simulink model "SIRAu_PI_vit"  (Simulink 8.7)
settings: Solver=ode5  StartTime=0.0  StopTime=Temps_manip  FixedStep=TE  RelTol=1e-3
values from neighbouring files (symbols this model uses):
  Kmes = 10.7e-3    (= 0.0107)    [Param_PI_Vit.m]
  Kp = Tn/Ti    (= 2.64498624343)    [Param_PI_Vit.m]    (also in labo4.m = wc * sqrt(1+(wc*tau_ele)^2) * Ti / K_total)
  Td = 0    [Param_PI_Vit.m]
  TE = 1e-3    (= 0.001)    [Param_PI_Vit.m]
  Ti = 2 * Ks * T2    (= 0.0030245904)    [Param_PI_Vit.m]    (also in labo4.m = 0.008)
libraries: xpcnilib x2, simulink x1, simulink_extras x1
settings Model: Creator=allenbach  LastModifiedBy=jeremy.olivier
settings SolverCC: EnableConcurrentExecution=on  PositivePriorityOrder=on  AutoInsertRateTranBlk=on
settings DataIOCC: LimitDataPoints=off  SignalLoggingSaveFormat=ModelDataLogs
settings OptimizationCC: BlockReduction=off  OptimizeBlockIOStorage=off  BufferReuse=off  GlobalBufferReuse=off  ExpressionFolding=off  ExpressionDepthLimit=2147483647  LocalBlockOutputs=off
settings DebuggingCC: SolverPrmCheckMsg=warning  FcnCallInpInsideContextMsg=UseLocalSettings  StateNameClashWarn=warning
settings HardwareCC: ProdIntDivRoundTo=Zero  ProdEndianess=LittleEndian  ProdLongLongMode=on  ProdHWDeviceType=Generic->32-bit x86 compatible
settings RTWCC: SystemTargetFile=slrt.tlc  TemplateMakefile=slrt_default_tmf  Description=Simulink Real-Time  RTWCompilerOptimization=on
settings SimulinkRealTimeCC: GeneratePreprocessorConditionals=Disable all  RL32LogBufSizeModifier=300000

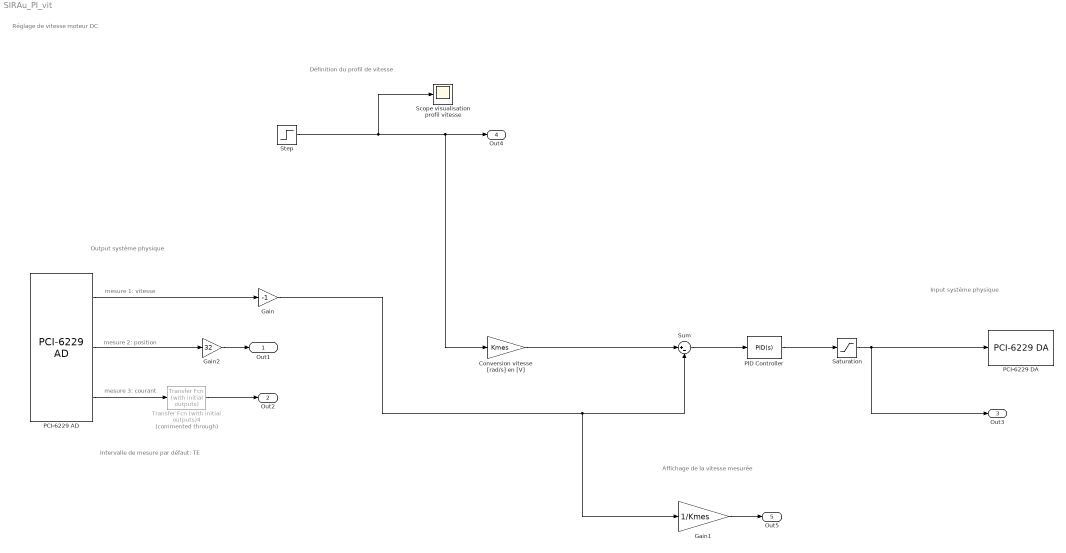
== system SIRAu_PI_vit ==
  note: Affichage de la vitesse mesurée
  note: Output système physique
  note: Input système physique
  note: Définition du profil de vitesse
  note: mesure 1: vitesse
  note: Réglage de vitesse moteur DC
  note: mesure 3: courant
  note: mesure 2: position
  note: Intervalle de mesure par défaut: TE
  Conversion vitesse [rad/s] en [V] : Gain  Gain=Kmes
  Gain : Gain  Gain=-1
  Gain1 : Gain  Gain=1/Kmes
  Gain2 : Gain  Gain=32
  PCI-6229 AD : xpcnilib/A//D/M Series/PCI-6229 AD  channel=[1,2,3]  range=[10]  coupling=[0]  scantime=5e-6  sampletime=TE  slot=-1
  PCI-6229 DA : xpcnilib/D//A/M Series/PCI-6229 DA  channel=[1]  reset=[1]  initValue=[0]  sampletime=TE  slot=-1
  PID Controller : simulink/Continuous/PID Controller  Controller=PID  TimeDomain=Continuous-time  SampleTime=-1  IntegratorMethod=Forward Euler  FilterMethod=Forward Euler  Form=Parallel  UseFilter=on  ControllerParametersSource=internal  P=Kp  I=1/Ti  D=Td  N=100  InitialConditionSource=internal  InitialConditionForIntegrator=0  InitialConditionForFilter=0  ExternalReset=none  LimitOutput=off  UpperSaturationLimit=inf  LowerSaturationLimit=-inf  LinearizeAsGain=on  AntiWindupMode=none  Kb=1  TrackingMode=off  Kt=1  PParamMin=[]  PParamMax=[]  IParamMin=[]  IParamMax=[]  DParamMin=[]  DParamMax=[]  NParamMin=[]  NParamMax=[]  KbParamMin=[]  KbParamMax=[]  KtParamMin=[]  KtParamMax=[]  POutMin=[]  POutMax=[]  IOutMin=[]  IOutMax=[]  DOutMin=[]  DOutMax=[]  NOutMin=[]  NOutMax=[]  KbOutMin=[]  KbOutMax=[]  KtOutMin=[]  KtOutMax=[]  IntegratorOutMin=[]  IntegratorOutMax=[]  FilterOutMin=[]  FilterOutMax=[]  SumOutMin=[]  SumOutMax=[]  SumI1OutMin=[]  SumI1OutMax=[]  SumI2OutMin=[]  SumI2OutMax=[]  SumI3OutMin=[]  SumI3OutMax=[]  SumDOutMin=[]  SumDOutMax=[]  SaturationOutMin=[]  SaturationOutMax=[]  IntegratorContinuousStateAttributes=''  IntegratorStateMustResolveToSignalObject=off  IntegratorRTWStateStorageClass=Auto  FilterContinuousStateAttributes=''  FilterStateMustResolveToSignalObject=off  FilterRTWStateStorageClass=Auto  DifferentiatorICPrevScaledInput=0  DifferentiatorOutMin=[]  DifferentiatorOutMax=[]
  Saturation : Saturate  UpperLimit=15  LowerLimit=-15
  Scope visualisation profil vitesse : Scope
  Step : Step  After=100  SampleTime=TE
  Sum : Sum  Inputs=|+-
  Transfer Fcn (with initial outputs)4 : simulink_extras/Additional Linear/Transfer Fcn (with initial outputs)  Commented=through  N=[1]  D="[0.002  1]"  Y0=0  U0=0
  Out1 : Outport
  Out2 : Outport  Port=2
  Out3 : Outport  Port=3
  Out4 : Outport  Port=4
  Out5 : Outport  Port=5
  wires:
  PCI-6229 AD/1 -> Gain/1
  PCI-6229 AD/3 -> Transfer Fcn (with initial outputs)4/1
  Transfer Fcn (with initial outputs)4/1 -> Out2/1
  PCI-6229 AD/2 -> Gain2/1
  Gain1/1 -> Out5/1
  Sum/1 -> PID Controller/1
  PID Controller/1 -> Saturation/1
  Step/1 -> Conversion vitesse [rad/s] en [V]/1, Out4/1, Scope visualisation profil vitesse/1
  Gain2/1 -> Out1/1
  Gain/1 -> Gain1/1, Sum/2
  Conversion vitesse [rad/s] en [V]/1 -> Sum/1
  Saturation/1 -> Out3/1, PCI-6229 DA/1
